simulink model "boeing747_longitudinal"  (R2021b)
settings: Solver=FixedStepAuto  StartTime=0.0  StopTime=30  FixedStep=1e-3  RelTol=1e-3
values from neighbouring files (symbols this model uses):
  planta = ss(A, B, C, D)    [obterPlantaLongitudinal.m]    (also in plotStepPlanta.m = obterPlantaLongitudinal())
undefined symbols (not defined in the file or in its folder): controlador, hr, varh
settings Model: Creator=mmaximo  LastModifiedBy=Eric
settings SolverCC: AlgebraicLoopSolver=TrustRegion
settings DebuggingCC: SFMachineParentedDataDiag=warning

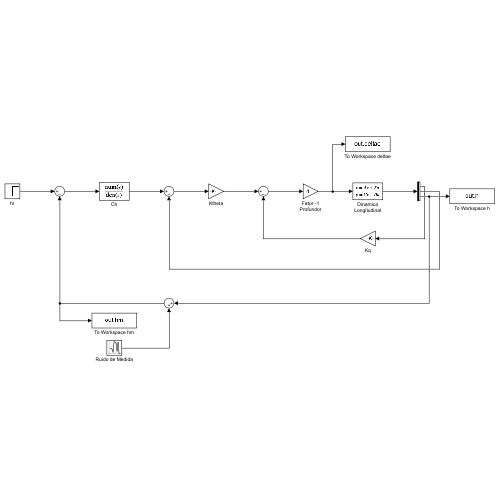
[thumbnail: Simulink's stored preview of the top-level diagram]
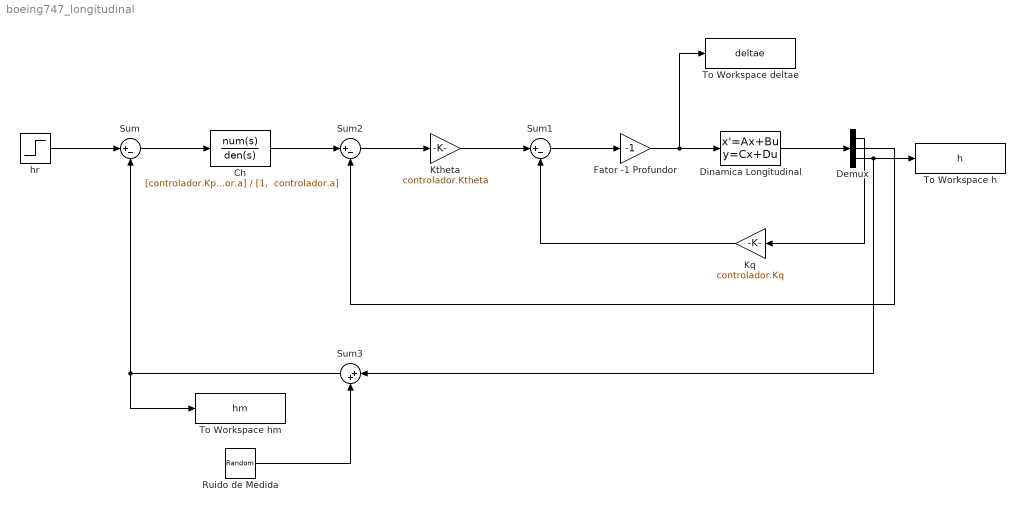
== system boeing747_longitudinal ==
  Ch : TransferFcn  Numerator=[controlador.Kph + controlador.Kdh * controlador.a, controlador.Kph * controlador.a]  Denominator="[1,  controlador.a]"
  Demux : Demux  Outputs=3
  Dinamica Longitudinal : StateSpace  A=planta.A  B=planta.B  C=planta.C  D=planta.D  InitialCondition=0
  Fator -1 Profundor : Gain  Gain=-1
  Kq : Gain  Gain=controlador.Kq
  Ktheta : Gain  Gain=controlador.Ktheta
  Ruido de Medida : RandomNumber  Variance=varh  SampleTime=1.0 / 100.0
  Sum : Sum  Inputs=|+-
  Sum1 : Sum  Inputs=|+-
  Sum2 : Sum  Inputs=|+-
  Sum3 : Sum  Inputs=|++
  To Workspace deltae : ToWorkspace  VariableName=deltae  SaveFormat=Structure With Time  SampleTime=-1
  To Workspace h : ToWorkspace  VariableName=h  SaveFormat=Structure With Time  SampleTime=-1
  To Workspace hm : ToWorkspace  VariableName=hm  SaveFormat=Structure With Time  SampleTime=-1
  hr : Step  Time=0  After=hr  SampleTime=0
  wires:
  Demux/3 -> Sum3/1, To Workspace h/1
  Sum2/1 -> Ktheta/1
  Ruido de Medida/1 -> Sum3/2
  Sum3/1 -> Sum/2, To Workspace hm/1
  hr/1 -> Sum/1
  Sum/1 -> Ch/1
  Ch/1 -> Sum2/1
  Dinamica Longitudinal/1 -> Demux/1
  Ktheta/1 -> Sum1/1
  Sum1/1 -> Fator -1 Profundor/1
  Fator -1 Profundor/1 -> To Workspace deltae/1, Dinamica Longitudinal/1
  Demux/2 -> Sum2/2
  Demux/1 -> Kq/1
  Kq/1 -> Sum1/2
